simulink model "grab_c_function"  (R2020b)
settings: Solver=VariableStepAuto  StartTime=0.0  StopTime=10.0  RelTol=1e-3
settings Model: Creator=shui  LastModifiedBy=shui
settings SFSimCC: CustomCodeGlobalsAsFunctionIO=on
settings SFSimCC: SimCustomHeaderCode=|
  | #include "adder.h"
  | #include "Simplex_full_v2_func.h"
settings SFSimCC: SimUserSources=|
  | adder.c
  | Simplex_full_v2_func.c

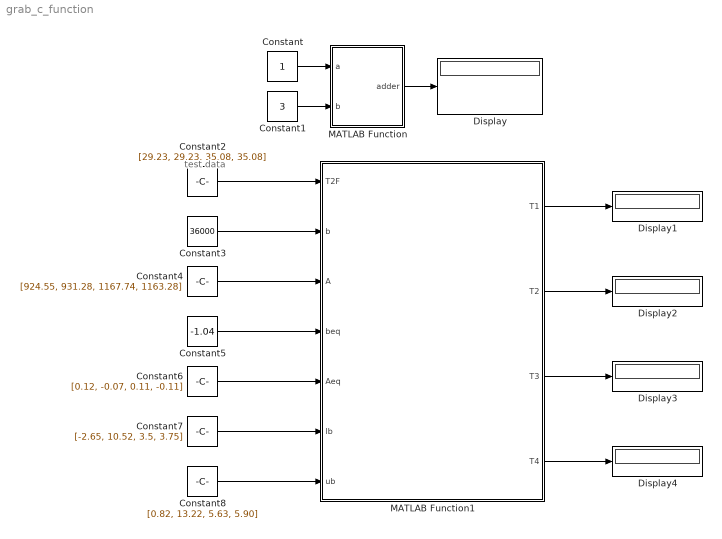
== system grab_c_function ==
  note: test data
  Constant : Constant
  Constant1 : Constant  Value=3
  Constant2 : Constant  Value=[29.23, 29.23, 35.08, 35.08]
  Constant3 : Constant  Value=36000
  Constant4 : Constant  Value=[924.55, 931.28, 1167.74, 1163.28]
  Constant5 : Constant  Value=-1.04
  Constant6 : Constant  Value=[0.12, -0.07, 0.11, -0.11]
  Constant7 : Constant  Value=[-2.65, 10.52, 3.5, 3.75]
  Constant8 : Constant  Value=[0.82, 13.22, 5.63, 5.90]
  Display{,1..4} (5 alike) : Display
      Display1 settings: Decimation=3
      Display2 settings: Decimation=3
      Display3 settings: Decimation=3
      Display4 settings: Decimation=3
  MATLAB Function : MATLAB Function  TreatAsAtomicUnit=on
  MATLAB Function1 : MATLAB Function  TreatAsAtomicUnit=on
  wires:
  MATLAB Function/1(adder) -> Display/1
  Constant/1 -> MATLAB Function/1(a)
  Constant1/1 -> MATLAB Function/2(b)
  Constant2/1 -> MATLAB Function1/1(T2F)
  Constant3/1 -> MATLAB Function1/2(b)
  Constant4/1 -> MATLAB Function1/3(A)
  Constant5/1 -> MATLAB Function1/4(beq)
  Constant6/1 -> MATLAB Function1/5(Aeq)
  Constant7/1 -> MATLAB Function1/6(lb)
  Constant8/1 -> MATLAB Function1/7(ub)
  MATLAB Function1/1(T1) -> Display1/1
  MATLAB Function1/2(T2) -> Display2/1
  MATLAB Function1/3(T3) -> Display3/1
  MATLAB Function1/4(T4) -> Display4/1

== matlab function grab_c_function/MATLAB Function1 ==
  data: T2F input; T1 output; b input; A input; beq input; Aeq input; lb input; ub input; T2 output; T3 output; T4 output
function [T1, T2, T3, T4] = call_simplex(T2F, b, A, beq, Aeq, lb, ub)

% T2F, A, Aeq, lb, ub:  [1 * 4] single (float) matrix
% b, A:                 single (float)

% force single instead of MATLAB defualt double
T1 = single(0);
T2 = single(0);
T3 = single(0);
T4 = single(0);
coder.cinclude("Simplex_full_v2_func.h");

% use pass by address to output T1, T2, T3, T4
coder.ceval("simplex_func", T2F(1), T2F(2), T2F(3), T2F(4), ...
                            b, A(1), A(2), A(3), A(4), ...
                            beq, Aeq(1), Aeq(2), Aeq(3), Aeq(4), ...
                            lb(1), lb(2), lb(3), lb(4), ...
                            ub(1), ub(2), ub(3), ub(4), ...
                            coder.ref(T1), coder.ref(T2), coder.ref(T3), coder.ref(T4));

end

== matlab function grab_c_function/MATLAB Function ==
  data: a input; adder output; b input
function adder  = fcn_test(a, b)
adder = 0;
coder.cinclude('adder.h');
adder = coder.ceval('adder', a, b);
end
